simulink model "Task7"  (R2023b)
settings: Solver=VariableStepAuto  StartTime=0.0  StopTime=1800  RelTol=1e-3
InitFcn:
  | run("Linear_Model.m")
values from neighbouring files (symbols this model uses):
  A_Lat = [Yv   Yp+w0   Yr-u0         gravity*cos(theta0)     0 ... (first row only)    [Linear_Model.m]
  A_Long = [Xu                    Xw                        -w0                            -gravity*cos(theta0) ... (first row only)    [Linear_Model.m]
  B_Lat = [Yda          Ydr ... (first row only)    [Linear_Model.m]
  B_Long = [Xde                         Xdth ... (first row only)    [Linear_Model.m]
  C_Lat = eye(5)    [Linear_Model.m]
  C_Long = eye(4)    [Linear_Model.m]
  D_Lat = zeros(5,2)    [Linear_Model.m]
  D_Long = zeros(4,2)    [Linear_Model.m]
  F_gravity_0 = mass*gravity*[sin(states_0(8)) ... (first row only)    [Data_edit.m]
  gravity = Airplane_data(52)    [Data_edit.m]
  Ixx = Airplane_data(53)    [Data_edit.m]
  Iyy = Airplane_data(54)    [Data_edit.m]
  Izz = Airplane_data(55)    [Data_edit.m]
  M0 = [0;0;0]    [Data_edit.m]
  mass = Airplane_data(51)    [Data_edit.m]
  Matrix_controls = [ 0             Xde             Xdth            0 ... (first row only)    [Data_edit.m]
  Matrix_states = [Xu   0   Xw  0   0   0   0 ... (first row only)    [Data_edit.m]
  p0 = states_0(4)    [Data_edit.m]
  phi0 = states_0(7)    [Data_edit.m]
  psi0 = states_0(9)    [Data_edit.m]
  q0 = states_0(5)    [Data_edit.m]
  r0 = states_0(6)    [Data_edit.m]
  states_0 = Airplane_data(4:15)    [Data_edit.m]
  theta0 = states_0(8)    [Data_edit.m]
  u0 = states_0(1)    [Data_edit.m]
  v0 = states_0(2)    [Data_edit.m]
  w0 = states_0(3)    [Data_edit.m]
undefined symbols (not defined in the file or in its folder): Earth, sigbuilder_block, WGS84
libraries: simulink_extras x35, cstblocks x17, slpidlib x12, aerolibasang x2, aerolibfltsims x2, shared6dof x1, dspsigops x1, aerolibtransform2 x1
(part 2 of 2)

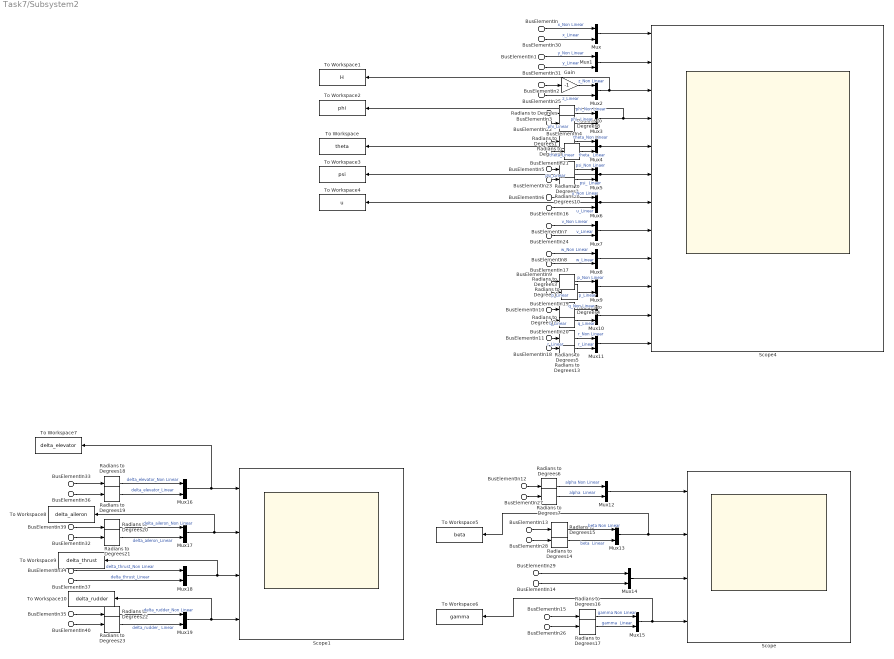
== system Task7/Subsystem2 ==
  BusElementIn16 : Inport  PortName=states_linear  Element=u
  BusElementIn17 : Inport  PortName=states_linear  Element=w
  BusElementIn18 : Inport  PortName=states_linear  Element=r
  BusElementIn19 : Inport  PortName=states_linear  Element=p
  BusElementIn20 : Inport  PortName=states_linear  Element=q
  BusElementIn21 : Inport  PortName=states_linear  Element=theta
  BusElementIn22 : Inport  PortName=states_linear  Element=phi
  BusElementIn23 : Inport  PortName=states_linear  Element=psi
  BusElementIn24 : Inport  PortName=states_linear  Element=v
  BusElementIn25 : Inport  PortName=states_linear  Element=H
  BusElementIn27 : Inport  PortName=states_linear  Element=alpha
  BusElementIn28 : Inport  PortName=states_linear  Element=beta
  BusElementIn29 : Inport  PortName=states_linear  Element=v_tot
  BusElementIn30 : Inport  PortName=states_linear  Element=x
  BusElementIn31 : Inport  PortName=states_linear  Element=y
  BusElementIn26 : Inport  PortName=states_linear  Element=gamma(rad)
  BusElementIn12 : Inport  Port=2  PortName=states  Element=alpha
  BusElementIn13 : Inport  Port=2  PortName=states  Element=betaa
  BusElementIn14 : Inport  Port=2  PortName=states  Element=v_tot
  BusElementIn : Inport  Port=2  PortName=states  Element=x
  BusElementIn1 : Inport  Port=2  PortName=states  Element=y
  BusElementIn2 : Inport  Port=2  PortName=states  Element=z
  BusElementIn3 : Inport  Port=2  PortName=states  Element=phi
  BusElementIn4 : Inport  Port=2  PortName=states  Element=ceta
  BusElementIn5 : Inport  Port=2  PortName=states  Element=psi
  BusElementIn6 : Inport  Port=2  PortName=states  Element=u
  BusElementIn7 : Inport  Port=2  PortName=states  Element=v
  BusElementIn8 : Inport  Port=2  PortName=states  Element=w
  BusElementIn9 : Inport  Port=2  PortName=states  Element=p
  BusElementIn10 : Inport  Port=2  PortName=states  Element=q
  BusElementIn11 : Inport  Port=2  PortName=states  Element=r
  BusElementIn15 : Inport  Port=2  PortName=states  Element=gamma
  BusElementIn32 : Inport  Port=3  PortName=Conrol Action Non Linear  Element=delta_aileron
  BusElementIn33 : Inport  Port=3  PortName=Conrol Action Non Linear  Element=delta_elevator
  BusElementIn34 : Inport  Port=3  PortName=Conrol Action Non Linear  Element=delta_thrust
  BusElementIn35 : Inport  Port=3  PortName=Conrol Action Non Linear  Element=delta_ruuder
  BusElementIn36 : Inport  Port=4  PortName="Conrol Action  Linear"  Element=Long_Control_Action.delta_elevator
  BusElementIn37 : Inport  Port=4  PortName="Conrol Action  Linear"  Element=Long_Control_Action.delta_thrust
  BusElementIn39 : Inport  Port=4  PortName="Conrol Action  Linear"  Element=Lat_Control_Action.delta_aileron
  BusElementIn40 : Inport  Port=4  PortName="Conrol Action  Linear"  Element=Lat_Control_Action.delta_ruuder
  Gain : Gain  Gain=-1
  Mux{,1..19} (20 alike) : Mux  Inputs=2
  Radians to Degrees{,1..23} (24 alike) : simulink_extras/Transformations/Radians to Degrees
  Scope : Scope  NumInputPorts=4
  Scope1 : Scope  NumInputPorts=4
  Scope4 : Scope  NumInputPorts=12
  To Workspace : ToWorkspace  VariableName=theta  SampleTime=-1
  To Workspace1 : ToWorkspace  VariableName=H  SampleTime=-1
  To Workspace10 : ToWorkspace  VariableName=delta_rudder  SampleTime=-1
  To Workspace2 : ToWorkspace  VariableName=phi  SampleTime=-1
  To Workspace3 : ToWorkspace  VariableName=psi  SampleTime=-1
  To Workspace4 : ToWorkspace  VariableName=u  SampleTime=-1
  To Workspace5 : ToWorkspace  VariableName=beta  SampleTime=-1
  To Workspace6 : ToWorkspace  VariableName=gamma  SampleTime=-1
  To Workspace7 : ToWorkspace  VariableName=delta_elevator  SampleTime=-1
  To Workspace8 : ToWorkspace  VariableName=delta_aileron  SampleTime=-1
  To Workspace9 : ToWorkspace  VariableName=delta_thrust  SampleTime=-1
  wires:
  BusElementIn1/1 -> Mux1/1  "y_Non Linear"
  BusElementIn/1 -> Mux/1  "x_Non Linear"
  Gain/1 -> Mux2/1  "z_Non Linear"
  BusElementIn2/1 -> Gain/1
  Mux/1 -> Scope4/1
  Mux1/1 -> Scope4/2
  Mux2/1 -> Scope4/3, To Workspace1/1
  BusElementIn4/1 -> Radians to Degrees1/1
  Radians to Degrees/1 -> Mux3/1  "phi_Non Linear"
  BusElementIn5/1 -> Radians to Degrees2/1
  Radians to Degrees1/1 -> Mux4/1  "theta_Non Linear"
  Radians to Degrees2/1 -> Mux5/1  "psi_Non Linaer"
  BusElementIn3/1 -> Radians to Degrees/1
  Mux5/1 -> To Workspace3/1, Scope4/6
  Mux4/1 -> To Workspace/1, Scope4/5
  Mux3/1 -> To Workspace2/1, Scope4/4
  Mux6/1 -> Scope4/7, To Workspace4/1
  Mux7/1 -> Scope4/8
  Mux8/1 -> Scope4/9
  BusElementIn6/1 -> Mux6/1  "u_Non Linear"
  BusElementIn7/1 -> Mux7/1  "v_Non Linear"
  BusElementIn8/1 -> Mux8/1  "w_Non Linear"
  Mux9/1 -> Scope4/10
  BusElementIn9/1 -> Radians to Degrees3/1
  Mux10/1 -> Scope4/11
  Mux11/1 -> Scope4/12
  BusElementIn10/1 -> Radians to Degrees4/1
  BusElementIn11/1 -> Radians to Degrees5/1
  Radians to Degrees3/1 -> Mux9/1  "p_Non Linear"
  Radians to Degrees4/1 -> Mux10/1  "q_Non Linear"
  Radians to Degrees5/1 -> Mux11/1  "r_Non Linear"
  BusElementIn30/1 -> Mux/2  "x_Linear"
  BusElementIn31/1 -> Mux1/2  "y_Linear"
  BusElementIn25/1 -> Mux2/2  "z_Linear"
  BusElementIn16/1 -> Mux6/2  "u_Linear"
  BusElementIn17/1 -> Mux8/2  "w_Linear"
  BusElementIn24/1 -> Mux7/2  "v_Linear"
  BusElementIn22/1 -> Radians to Degrees8/1  "phi_Linear"
  BusElementIn21/1 -> Radians to Degrees9/1  "theta_Linear"
  BusElementIn23/1 -> Radians to Degrees10/1  "psi_Linear"
  BusElementIn19/1 -> Radians to Degrees11/1  "p_Linear"
  BusElementIn20/1 -> Radians to Degrees12/1  "q_Linear"
  BusElementIn18/1 -> Radians to Degrees13/1  "r_Linear"
  Mux12/1 -> Scope/1
  BusElementIn12/1 -> Radians to Degrees6/1
  Radians to Degrees6/1 -> Mux12/1  "alpha Non Linear"
  Radians to Degrees7/1 -> Mux12/2  "alpha  Linear"
  BusElementIn27/1 -> Radians to Degrees7/1
  Mux13/1 -> To Workspace5/1, Scope/2
  Radians to Degrees8/1 -> Mux3/2  "phi_ Linear"
  Radians to Degrees9/1 -> Mux4/2  "theta_ Linear"
  Radians to Degrees10/1 -> Mux5/2  "psi_ Linaer"
  Radians to Degrees11/1 -> Mux9/2  "p_Linear"
  Radians to Degrees12/1 -> Mux10/2  "q_Linear"
  Radians to Degrees13/1 -> Mux11/2  "r_Linear"
  BusElementIn28/1 -> Radians to Degrees14/1
  Radians to Degrees14/1 -> Mux13/2  "beta  Linear"
  BusElementIn13/1 -> Radians to Degrees15/1
  Radians to Degrees15/1 -> Mux13/1  "beta Non Linear"
  Mux14/1 -> Scope/3
  BusElementIn14/1 -> Mux14/2
  BusElementIn29/1 -> Mux14/1
  BusElementIn15/1 -> Radians to Degrees16/1
  BusElementIn26/1 -> Radians to Degrees17/1
  Radians to Degrees16/1 -> Mux15/1  "gamma Non Linear"
  Radians to Degrees17/1 -> Mux15/2  "gamma  Linear"
  Mux16/1 -> To Workspace7/1, Scope1/1
  Mux17/1 -> To Workspace8/1, Scope1/2
  Mux18/1 -> To Workspace9/1, Scope1/3
  Mux19/1 -> To Workspace10/1, Scope1/4
  BusElementIn36/1 -> Radians to Degrees19/1
  BusElementIn33/1 -> Radians to Degrees18/1
  BusElementIn39/1 -> Radians to Degrees20/1
  BusElementIn32/1 -> Radians to Degrees21/1
  BusElementIn34/1 -> Mux18/1  "delta_thrust_Non Linear"
  BusElementIn37/1 -> Mux18/2  "delta_thrust_Linear"
  BusElementIn40/1 -> Radians to Degrees23/1
  BusElementIn35/1 -> Radians to Degrees22/1
  Radians to Degrees18/1 -> Mux16/1  "delta_elevator_Non Linear"
  Radians to Degrees19/1 -> Mux16/2  "delta_elevator_Linear"
  Radians to Degrees20/1 -> Mux17/1  "delta_aileron_Non Linear"
  Radians to Degrees21/1 -> Mux17/2  "delta_aileron_Linear"
  Radians to Degrees22/1 -> Mux19/1  "delta_rudder_Non Linear"
  Radians to Degrees23/1 -> Mux19/2  "delta_rudder_ Linear"
  Mux15/1 -> To Workspace6/1, Scope/4

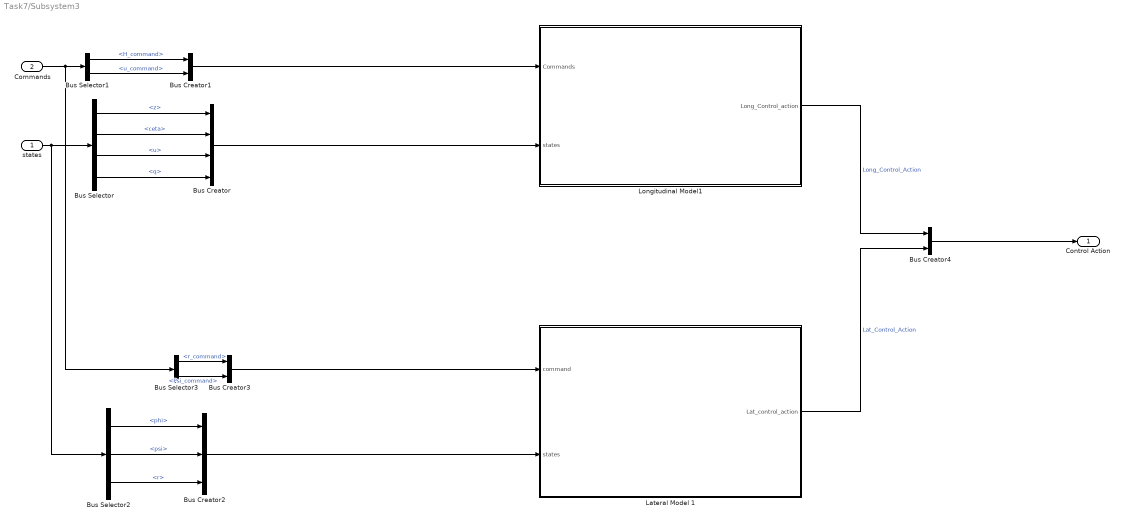
== system Task7/Subsystem3 ==
  states : Inport
  Commands : Inport  Port=2
  Bus Creator : BusCreator  Inputs=4
  Bus Creator1 : BusCreator  Inputs=2
  Bus Creator2 : BusCreator  Inputs=3
  Bus Creator3 : BusCreator  Inputs=2
  Bus Creator4 : BusCreator  Inputs=2
  Bus Selector : BusSelector  OutputSignals=z,ceta,u,q
  Bus Selector1 : BusSelector  OutputSignals=H_command,u_command
  Bus Selector2 : BusSelector  OutputSignals=phi,psi,r
  Bus Selector3 : BusSelector  OutputSignals=r_command,Psi_command
  Lateral Model 1 : Subsystem
  Longitudinal Model1 : Subsystem
  Control Action : Outport
  wires:
  states/1 -> Bus Selector2/1, Bus Selector/1
  Bus Selector/4 -> Bus Creator/4  "<q>"
  Bus Selector/3 -> Bus Creator/3  "<u>"
  Bus Selector/2 -> Bus Creator/2  "<ceta>"
  Bus Selector/1 -> Bus Creator/1  "<z>"
  Bus Creator/1 -> Longitudinal Model1/2(states)
  Commands/1 -> Bus Selector3/1, Bus Selector1/1
  Bus Selector1/1 -> Bus Creator1/1  "<H_command>"
  Bus Selector1/2 -> Bus Creator1/2  "<u_command>"
  Bus Creator1/1 -> Longitudinal Model1/1(Commands)
  Bus Selector2/1 -> Bus Creator2/1  "<phi>"
  Bus Selector2/2 -> Bus Creator2/2  "<psi>"
  Bus Selector2/3 -> Bus Creator2/3  "<r>"
  Bus Creator2/1 -> Lateral Model 1/2(states)
  Bus Creator3/1 -> Lateral Model 1/1(command)
  Bus Selector3/1 -> Bus Creator3/1  "<r_command>"
  Bus Selector3/2 -> Bus Creator3/2  "<Psi_command>"
  Longitudinal Model1/1(Long_Control_action) -> Bus Creator4/1  "Long_Control_Action"
  Lateral Model 1/1(Lat_control_action) -> Bus Creator4/2  "Lat_Control_Action"
  Bus Creator4/1 -> Control Action/1

== system Task7/Subsystem4 ==
  States : Inport
  Bus Selector1 : BusSelector  OutputSignals=x,y,z,phi,ceta,psi
  Demux : Demux  Outputs=2
  Flat Earth to LLA : aerolibtransform2/Flat Earth to LLA  units=Metric (MKS)  ptype=Earth (WGS84)  F=1/298.257223563  R=6378137  refPosPort=off  LL0=[0 10]  psi=0
  FlightGear Preconfigured 6DoF Animation : aerolibfltsims/FlightGear Preconfigured 6DoF Animation  xFlightGearVersion=v2019.1  DestinationIpAddress=127.0.0.1  DestinationPort=5502  SampleTime=1/30  packetVersion=24
  Generate Run Script : aerolibfltsims/Generate Run Script  Architecture=Win64  dataFlow=Send  GeometryModelName=c172p  AirportId=KSFO  RunwayId=10L  InitialAltitude=0  InitialHeading=0  OffsetDistance=0  OffsetAzimuth=0  InstallScenery=off  DisableShaders=on  OriginAddress=127.0.0.1  DestinationPort=5502  OriginPort=5505  LocalAddress=127.0.0.1  OutputFileName=runfg.bat  FlightGearBaseDirectory=C:\Program Files\FlightGear 2020.3
  Ground : Ground
  Mux : Mux  Inputs=3
  Mux1 : Mux  Inputs=3
  Mux2 : Mux
  wires:
  Mux1/1 -> Mux2/4
  Mux2/1 -> FlightGear Preconfigured 6DoF Animation/1
  Bus Selector1/6 -> Mux1/3  "<psi>"
  Flat Earth to LLA/1 -> Demux/1
  Bus Selector1/2 -> Mux/2  "<y>"
  Ground/1 -> Flat Earth to LLA/2
  Demux/1 -> Mux2/2
  Bus Selector1/5 -> Mux1/2  "<ceta>"
  Flat Earth to LLA/2 -> Mux2/3
  Mux/1 -> Flat Earth to LLA/1
  Bus Selector1/4 -> Mux1/1  "<phi>"
  Bus Selector1/3 -> Mux/3  "<z>"
  Bus Selector1/1 -> Mux/1  "<x>"
  Demux/2 -> Mux2/1
  States/1 -> Bus Selector1/1

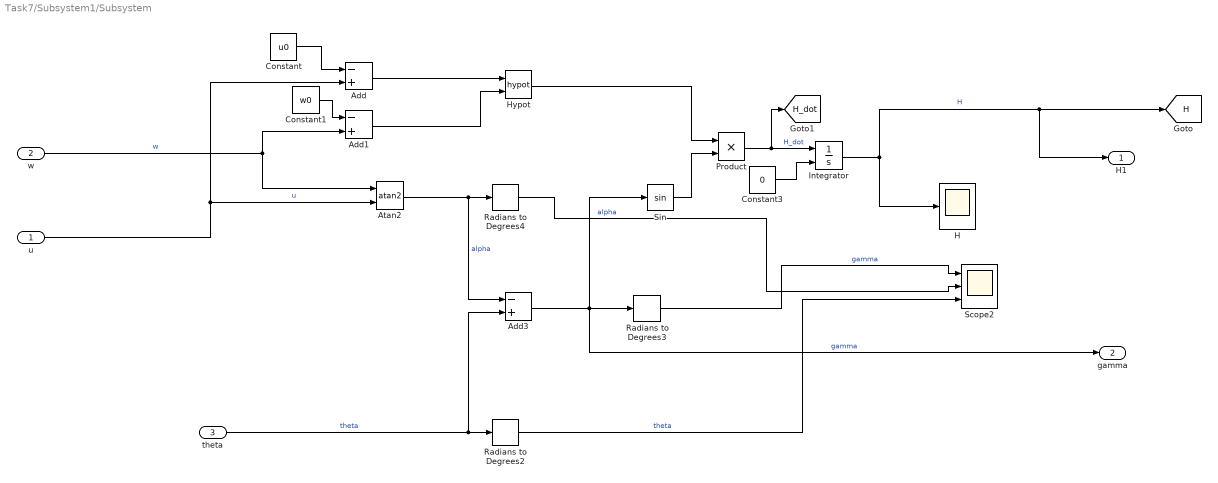
== system Task7/Subsystem1/Subsystem ==
  u : Inport
  w : Inport  Port=2
  theta : Inport  Port=3
  Add : Sum  Inputs=-+
  Add1 : Sum  Inputs=-+
  Add3 : Sum  Inputs=-+
  Atan2 : Trigonometry  Operator=atan2
  Constant : Constant  Value=u0
  Constant1 : Constant  Value=w0
  Constant3 : Constant  Value=0
  H : Scope
  Hypot : Math  Operator=hypot
  Integrator : Integrator  InitialConditionSource=external  InitialCondition=-states_0(12)
  Product : Product
  Radians to Degrees2 : simulink_extras/Transformations/Radians to Degrees
  Radians to Degrees3 : simulink_extras/Transformations/Radians to Degrees
  Radians to Degrees4 : simulink_extras/Transformations/Radians to Degrees
  Scope2 : Scope  NumInputPorts=3
  Sin : Trigonometry
  H1 : Outport
  gamma : Outport  Port=2
  tag scope: H=global, H_dot=global
  wires:
  Product/1 -> [H_dot], Integrator/1  "H_dot"
  Add3/1 -> gamma/1, Sin/1, Radians to Degrees3/1  "gamma"
  theta/1 -> Add3/2, Radians to Degrees2/1  "theta"
  Sin/1 -> Product/2
  Atan2/1 -> Radians to Degrees4/1, Add3/1  "alpha"
  Radians to Degrees4/1 -> Scope2/2  "alpha"
  Radians to Degrees2/1 -> Scope2/3  "theta"
  Radians to Degrees3/1 -> Scope2/1  "gamma"
  Integrator/1 -> H1/1, [H], H/1  "H"
  Hypot/1 -> Product/1
  Constant3/1 -> Integrator/2
  u/1 -> Add/2, Atan2/2  "u"
  w/1 -> Atan2/1, Add1/2  "w"
  Constant/1 -> Add/1
  Add/1 -> Hypot/1
  Constant1/1 -> Add1/1
  Add1/1 -> Hypot/2

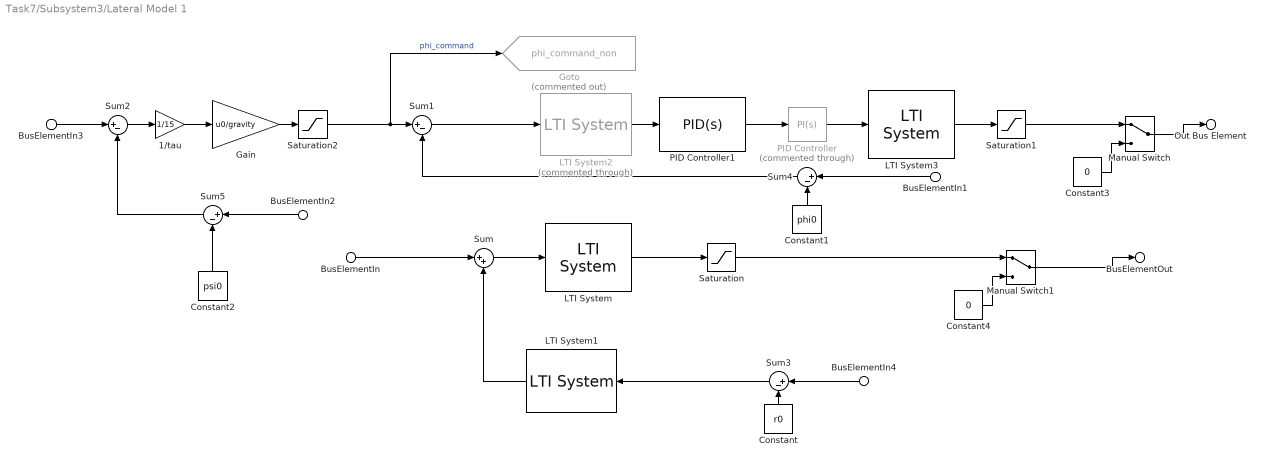
== system Task7/Subsystem3/Lateral Model 1 ==
  BusElementIn : Inport  PortName=command  Element=r_command
  BusElementIn3 : Inport  PortName=command  Element=Psi_command
  BusElementIn1 : Inport  Port=2  PortName=states  Element=phi
  BusElementIn2 : Inport  Port=2  PortName=states  Element=psi
  BusElementIn4 : Inport  Port=2  PortName=states  Element=r
  1/tau : Gain  Gain=1/15
  Constant : Constant  Value=r0
  Constant1 : Constant  Value=phi0
  Constant2 : Constant  Value=psi0
  Constant3 : Constant  Value=0
  Constant4 : Constant  Value=0
  Gain : Gain  Gain=u0/gravity
  Goto : Goto  Commented=on  GotoTag=phi_command_non  TagVisibility=global
  LTI System : cstblocks/LTI System  sys=servo  IC=[]  PadeOrder=0
  LTI System1 : cstblocks/LTI System  sys=HPF_Washout  IC=[]  PadeOrder=0
  LTI System2 : cstblocks/LTI System  Commented=through  sys=Roll_Comp  IC=[]  PadeOrder=0
  LTI System3 : cstblocks/LTI System  sys=servo  IC=[]  PadeOrder=0
  Manual Switch : ManualSwitch
  Manual Switch1 : ManualSwitch
  PID Controller : slpidlib/PID Controller  Commented=through  Controller=PI  Form=Parallel  TimeDomain=Continuous-time  UseExternalTs=off  SampleTime=-1  IntegratorMethod=Forward Euler  FilterMethod=Forward Euler  ControllerParametersSource=internal  P=1.6  I=.0254  UseKiTs=off  D=0  N=100  UseFilter=on  TunerSelectOption=Transfer Function Based (PID Tuner App)  InitialConditionSource=internal  InitialConditionForIntegrator=0  InitialConditionForFilter=0  DifferentiatorICPrevScaledInput=0  ExternalReset=none  TrackingMode=off  Kt=1  LimitOutput=off  SatLimitsSource=internal  UpperSaturationLimit=inf  LowerSaturationLimit=-inf  LinearizeAsGain=on  AntiWindupMode=none  Kb=1  LimitIntegrator=off  UpperIntegratorSaturationLimit=inf  LowerIntegratorSaturationLimit=-inf  POutMin=[]  POutMax=[]  IOutMin=[]  IOutMax=[]  DOutMin=[]  DOutMax=[]  NOutMin=[]  NOutMax=[]  SumOutMin=[]  SumOutMax=[]  SaturationOutMin=[]  SaturationOutMax=[]  PParamMin=[]  PParamMax=[]  IParamMin=[]  IParamMax=[]  DParamMin=[]  DParamMax=[]  NParamMin=[]  NParamMax=[]  KbParamMin=[]  KbParamMax=[]  KtParamMin=[]  KtParamMax=[]  KbOutMin=[]  KbOutMax=[]  KtOutMin=[]  KtOutMax=[]  IntegratorOutMin=[]  IntegratorOutMax=[]  FilterOutMin=[]  FilterOutMax=[]  SumI1OutMin=[]  SumI1OutMax=[]  SumI2OutMin=[]  SumI2OutMax=[]  SumI3OutMin=[]  SumI3OutMax=[]  SumI4OutMin=[]  SumI4OutMax=[]  SumDOutMin=[]  SumDOutMax=[]  DifferentiatorOutMin=[]  DifferentiatorOutMax=[]  FilterDiffOutCoefMin=[]  FilterDiffOutCoefMax=[]  ReciprocalOutMin=[]  ReciprocalOutMax=[]  SumDenOutMin=[]  SumDenOutMax=[]  SumNumOutMin=[]  SumNumOutMax=[]  DivideOutMin=[]  DivideOutMax=[]  UdiffTsProdOutMin=[]  UdiffTsProdOutMax=[]  NTsProdOutMin=[]  NTsProdOutMax=[]  UintegralTsProdOutMin=[]  UintegralTsProdOutMax=[]  UngainTsProdOutMin=[]  UngainTsProdOutMax=[]  ClampingZeroOutDataTypeStr=Inherit: Inherit via back propagation  ClampingZeroOutMin=[]  ClampingZeroOutMax=[]  FilterDenConstantOutDataTypeStr=Inherit: Inherit via back propagation  FilterDenConstantOutMin=[]  FilterDenConstantOutMax=[]  PCopyOutDataTypeStr=Inherit: Inherit via back propagation  PCopyOutMin=[]  PCopyOutMax=[]  NCopyOutDataTypeStr=Inherit: Inherit via back propagation  NCopyOutMin=[]  NCopyOutMax=[]  IntegratorContinuousStateAttributes=''  IntegratorStateMustResolveToSignalObject=off  IntegratorRTWStateStorageClass=Auto  FilterContinuousStateAttributes=''  FilterStateMustResolveToSignalObject=off  FilterRTWStateStorageClass=Auto  ParallelPVariant=InternalParameters  IdealPVariant=Disabled  IVariant=InternalParameters  DVariant=Disabled  IntegratorVariant=Continuous  SatVariant=Disabled  AWVariant=Passthrough  PCopyVariant=Disabled  TRVariant=Disabled  FdbkBlocksVariant=Forward  IdealPFdbkVariant=Disabled  SatFdbkVariant=Disabled  DerivativeFilterVariant=Disabled  NVariant=Disabled  NCopyVariant=Disabled_SignalSpec  FilterICVariant=Disabled  IntegratorICVariant=InternalICs  ExternalResetVariant=Disabled  TRSumVariant=Passthrough  SumFdbkVariant=Disabled  SumVariant=Sum_PI  TsampFilterVariant=InternalTs  TsampNgainVariant=Passthrough  TsampIntegralVariant=Disabled_SignalSpec  ExternalSaturationOutDataTypeStr=Inherit: Same as second input
  PID Controller1 : slpidlib/PID Controller  Controller=PID  Form=Parallel  TimeDomain=Continuous-time  UseExternalTs=off  SampleTime=-1  IntegratorMethod=Forward Euler  FilterMethod=Forward Euler  ControllerParametersSource=internal  P=3.4  I=0.05  UseKiTs=off  D=0.85  N=100  UseFilter=on  TunerSelectOption=Transfer Function Based (PID Tuner App)  InitialConditionSource=internal  InitialConditionForIntegrator=0  InitialConditionForFilter=0  DifferentiatorICPrevScaledInput=0  ExternalReset=none  TrackingMode=off  Kt=1  LimitOutput=off  SatLimitsSource=internal  UpperSaturationLimit=inf  LowerSaturationLimit=-inf  LinearizeAsGain=on  AntiWindupMode=none  Kb=1  LimitIntegrator=off  UpperIntegratorSaturationLimit=inf  LowerIntegratorSaturationLimit=-inf  POutMin=[]  POutMax=[]  IOutMin=[]  IOutMax=[]  DOutMin=[]  DOutMax=[]  NOutMin=[]  NOutMax=[]  SumOutMin=[]  SumOutMax=[]  SaturationOutMin=[]  SaturationOutMax=[]  PParamMin=[]  PParamMax=[]  IParamMin=[]  IParamMax=[]  DParamMin=[]  DParamMax=[]  NParamMin=[]  NParamMax=[]  KbParamMin=[]  KbParamMax=[]  KtParamMin=[]  KtParamMax=[]  KbOutMin=[]  KbOutMax=[]  KtOutMin=[]  KtOutMax=[]  IntegratorOutMin=[]  IntegratorOutMax=[]  FilterOutMin=[]  FilterOutMax=[]  SumI1OutMin=[]  SumI1OutMax=[]  SumI2OutMin=[]  SumI2OutMax=[]  SumI3OutMin=[]  SumI3OutMax=[]  SumI4OutMin=[]  SumI4OutMax=[]  SumDOutMin=[]  SumDOutMax=[]  DifferentiatorOutMin=[]  DifferentiatorOutMax=[]  FilterDiffOutCoefMin=[]  FilterDiffOutCoefMax=[]  ReciprocalOutMin=[]  ReciprocalOutMax=[]  SumDenOutMin=[]  SumDenOutMax=[]  SumNumOutMin=[]  SumNumOutMax=[]  DivideOutMin=[]  DivideOutMax=[]  UdiffTsProdOutMin=[]  UdiffTsProdOutMax=[]  NTsProdOutMin=[]  NTsProdOutMax=[]  UintegralTsProdOutMin=[]  UintegralTsProdOutMax=[]  UngainTsProdOutMin=[]  UngainTsProdOutMax=[]  ClampingZeroOutDataTypeStr=Inherit: Inherit via back propagation  ClampingZeroOutMin=[]  ClampingZeroOutMax=[]  FilterDenConstantOutDataTypeStr=Inherit: Inherit via back propagation  FilterDenConstantOutMin=[]  FilterDenConstantOutMax=[]  PCopyOutDataTypeStr=Inherit: Inherit via back propagation  PCopyOutMin=[]  PCopyOutMax=[]  NCopyOutDataTypeStr=Inherit: Inherit via back propagation  NCopyOutMin=[]  NCopyOutMax=[]  IntegratorContinuousStateAttributes=''  IntegratorStateMustResolveToSignalObject=off  IntegratorRTWStateStorageClass=Auto  FilterContinuousStateAttributes=''  FilterStateMustResolveToSignalObject=off  FilterRTWStateStorageClass=Auto  ParallelPVariant=InternalParameters  IdealPVariant=Disabled  IVariant=InternalParameters  DVariant=InternalParameters  IntegratorVariant=Continuous  SatVariant=Disabled  AWVariant=Passthrough  PCopyVariant=Disabled  TRVariant=Disabled  FdbkBlocksVariant=Forward  IdealPFdbkVariant=Disabled  SatFdbkVariant=Disabled  DerivativeFilterVariant=ContFilter  NVariant=InternalParameters  NCopyVariant=Disabled  FilterICVariant=InternalICsFilter  IntegratorICVariant=InternalICs  ExternalResetVariant=Disabled  TRSumVariant=Passthrough  SumFdbkVariant=Disabled  SumVariant=Sum_PID  TsampFilterVariant=InternalTs  TsampNgainVariant=Passthrough  TsampIntegralVariant=Disabled_SignalSpec  ExternalSaturationOutDataTypeStr=Inherit: Same as second input
  Saturation : Saturate  UpperLimit=deg2rad(30)  LowerLimit=deg2rad(-30)
  Saturation1 : Saturate  UpperLimit=deg2rad(50)  LowerLimit=deg2rad(-50)
  Saturation2 : Saturate  UpperLimit=deg2rad(30)  LowerLimit=deg2rad(-30)
  Sum : Sum  Inputs=|++
  Sum{1..5} (5 alike) : Sum  Inputs=|+-
  Out Bus Element : Outport  PortName=Lat_control_action  Element=delta_aileron
  BusElementOut : Outport  PortName=Lat_control_action  Element=delta_ruuder
  wires:
  Saturation2/1 -> Sum1/1, Goto/1  "phi_command"
  1/tau/1 -> Gain/1
  BusElementIn3/1 -> Sum2/1
  Sum2/1 -> 1/tau/1
  Gain/1 -> Saturation2/1
  Sum5/1 -> Sum2/2
  PID Controller1/1 -> PID Controller/1
  LTI System2/1 -> PID Controller1/1
  PID Controller/1 -> LTI System3/1
  LTI System3/1 -> Saturation1/1
  Sum1/1 -> LTI System2/1
  Sum4/1 -> Sum1/2
  LTI System1/1 -> Sum/2
  Sum3/1 -> LTI System1/1
  LTI System/1 -> Saturation/1
  Sum/1 -> LTI System/1
  BusElementIn/1 -> Sum/1
  Constant/1 -> Sum3/2
  BusElementIn1/1 -> Sum4/1
  Constant1/1 -> Sum4/2
  Constant2/1 -> Sum5/2
  BusElementIn4/1 -> Sum3/1
  BusElementIn2/1 -> Sum5/1
  Constant3/1 -> Manual Switch/2
  Saturation1/1 -> Manual Switch/1
  Manual Switch/1 -> Out Bus Element/1
  Constant4/1 -> Manual Switch1/2
  Saturation/1 -> Manual Switch1/1
  Manual Switch1/1 -> BusElementOut/1

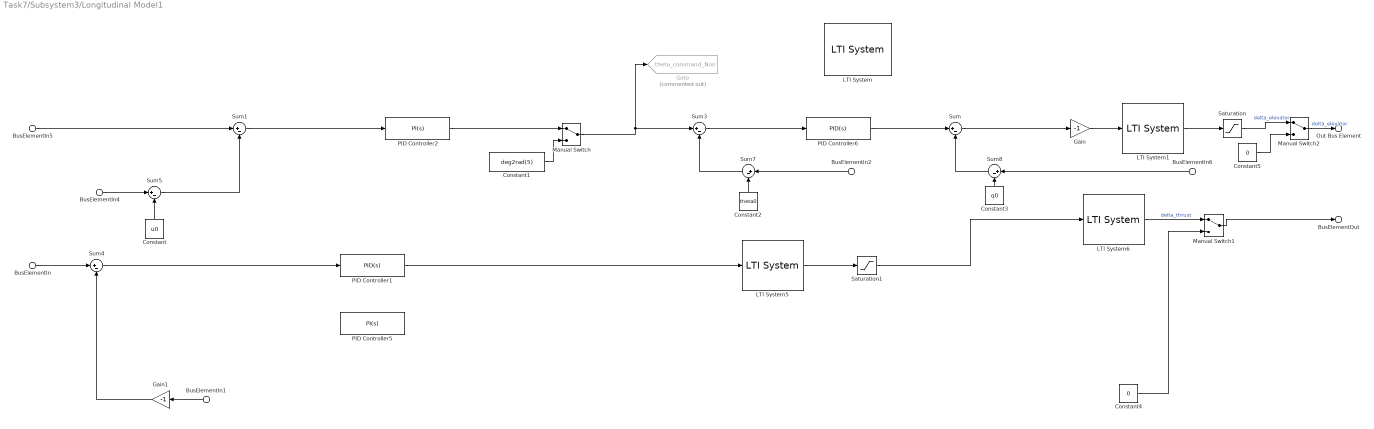
== system Task7/Subsystem3/Longitudinal Model1 ==
  BusElementIn5 : Inport  PortName=Commands  Element=u_command
  BusElementIn : Inport  PortName=Commands  Element=H_command
  BusElementIn1 : Inport  Port=2  PortName=states  Element=z
  BusElementIn4 : Inport  Port=2  PortName=states  Element=u
  BusElementIn2 : Inport  Port=2  PortName=states  Element=ceta
  BusElementIn6 : Inport  Port=2  PortName=states  Element=q
  Constant : Constant  Value=u0
  Constant1 : Constant  Value=deg2rad(5)
  Constant2 : Constant  Value=theta0
  Constant3 : Constant  Value=q0
  Constant4 : Constant  Value=0
  Constant5 : Constant  Value=0
  Gain : Gain  Gain=-1
  Gain1 : Gain  Gain=-1
  Goto : Goto  Commented=on  GotoTag=theta_command_Non  TagVisibility=global
  LTI System : cstblocks/LTI System  sys=PI_Pitch  IC=[]  PadeOrder=0
  LTI System1 : cstblocks/LTI System  sys=servo  IC=[]  PadeOrder=0
  LTI System5 : cstblocks/LTI System  sys=servo  IC=[]  PadeOrder=0
  LTI System6 : cstblocks/LTI System  sys=Engine_Lag  IC=[]  PadeOrder=0
  Manual Switch : ManualSwitch
  Manual Switch1 : ManualSwitch
  Manual Switch2 : ManualSwitch
  PID Controller1 : slpidlib/PID Controller  Controller=PID  Form=Parallel  TimeDomain=Continuous-time  UseExternalTs=off  SampleTime=-1  IntegratorMethod=Forward Euler  FilterMethod=Forward Euler  ControllerParametersSource=internal  P=88.8006309428434  I=0.0929360693607998  UseKiTs=off  D=2265.07533682159  N=14.0545983355681  UseFilter=on  TunerSelectOption=Transfer Function Based (PID Tuner App)  InitialConditionSource=internal  InitialConditionForIntegrator=0  InitialConditionForFilter=0  DifferentiatorICPrevScaledInput=0  ExternalReset=none  TrackingMode=off  Kt=1  LimitOutput=off  SatLimitsSource=internal  UpperSaturationLimit=inf  LowerSaturationLimit=-inf  LinearizeAsGain=on  AntiWindupMode=none  Kb=1  LimitIntegrator=off  UpperIntegratorSaturationLimit=inf  LowerIntegratorSaturationLimit=-inf  POutMin=[]  POutMax=[]  IOutMin=[]  IOutMax=[]  DOutMin=[]  DOutMax=[]  NOutMin=[]  NOutMax=[]  SumOutMin=[]  SumOutMax=[]  SaturationOutMin=[]  SaturationOutMax=[]  PParamMin=[]  PParamMax=[]  IParamMin=[]  IParamMax=[]  DParamMin=[]  DParamMax=[]  NParamMin=[]  NParamMax=[]  KbParamMin=[]  KbParamMax=[]  KtParamMin=[]  KtParamMax=[]  KbOutMin=[]  KbOutMax=[]  KtOutMin=[]  KtOutMax=[]  IntegratorOutMin=[]  IntegratorOutMax=[]  FilterOutMin=[]  FilterOutMax=[]  SumI1OutMin=[]  SumI1OutMax=[]  SumI2OutMin=[]  SumI2OutMax=[]  SumI3OutMin=[]  SumI3OutMax=[]  SumI4OutMin=[]  SumI4OutMax=[]  SumDOutMin=[]  SumDOutMax=[]  DifferentiatorOutMin=[]  DifferentiatorOutMax=[]  FilterDiffOutCoefMin=[]  FilterDiffOutCoefMax=[]  ReciprocalOutMin=[]  ReciprocalOutMax=[]  SumDenOutMin=[]  SumDenOutMax=[]  SumNumOutMin=[]  SumNumOutMax=[]  DivideOutMin=[]  DivideOutMax=[]  UdiffTsProdOutMin=[]  UdiffTsProdOutMax=[]  NTsProdOutMin=[]  NTsProdOutMax=[]  UintegralTsProdOutMin=[]  UintegralTsProdOutMax=[]  UngainTsProdOutMin=[]  UngainTsProdOutMax=[]  ClampingZeroOutDataTypeStr=Inherit: Inherit via back propagation  ClampingZeroOutMin=[]  ClampingZeroOutMax=[]  FilterDenConstantOutDataTypeStr=Inherit: Inherit via back propagation  FilterDenConstantOutMin=[]  FilterDenConstantOutMax=[]  PCopyOutDataTypeStr=Inherit: Inherit via back propagation  PCopyOutMin=[]  PCopyOutMax=[]  NCopyOutDataTypeStr=Inherit: Inherit via back propagation  NCopyOutMin=[]  NCopyOutMax=[]  IntegratorContinuousStateAttributes=''  IntegratorStateMustResolveToSignalObject=off  IntegratorRTWStateStorageClass=Auto  FilterContinuousStateAttributes=''  FilterStateMustResolveToSignalObject=off  FilterRTWStateStorageClass=Auto  ParallelPVariant=InternalParameters  IdealPVariant=Disabled  IVariant=InternalParameters  DVariant=InternalParameters  IntegratorVariant=Continuous  SatVariant=Disabled  AWVariant=Passthrough  PCopyVariant=Disabled  TRVariant=Disabled  FdbkBlocksVariant=Forward  IdealPFdbkVariant=Disabled  SatFdbkVariant=Disabled  DerivativeFilterVariant=ContFilter  NVariant=InternalParameters  NCopyVariant=Disabled  FilterICVariant=InternalICsFilter  IntegratorICVariant=InternalICs  ExternalResetVariant=Disabled  TRSumVariant=Passthrough  SumFdbkVariant=Disabled  SumVariant=Sum_PID  TsampFilterVariant=InternalTs  TsampNgainVariant=Passthrough  TsampIntegralVariant=Disabled_SignalSpec  ExternalSaturationOutDataTypeStr=Inherit: Same as second input
  PID Controller2 : slpidlib/PID Controller  Controller=PI  Form=Parallel  TimeDomain=Continuous-time  UseExternalTs=off  SampleTime=-1  IntegratorMethod=Forward Euler  FilterMethod=Forward Euler  ControllerParametersSource=internal  P=-0.0029780732187298  I=-6.00662195955179e-05  UseKiTs=off  D=-0.0901078465434796  N=4.30153629977803  UseFilter=on  TunerSelectOption=Transfer Function Based (PID Tuner App)  InitialConditionSource=internal  InitialConditionForIntegrator=0  InitialConditionForFilter=0  DifferentiatorICPrevScaledInput=0  ExternalReset=none  TrackingMode=off  Kt=1  LimitOutput=off  SatLimitsSource=internal  UpperSaturationLimit=inf  LowerSaturationLimit=-inf  LinearizeAsGain=on  AntiWindupMode=none  Kb=1  LimitIntegrator=off  UpperIntegratorSaturationLimit=inf  LowerIntegratorSaturationLimit=-inf  POutMin=[]  POutMax=[]  IOutMin=[]  IOutMax=[]  DOutMin=[]  DOutMax=[]  NOutMin=[]  NOutMax=[]  SumOutMin=[]  SumOutMax=[]  SaturationOutMin=[]  SaturationOutMax=[]  PParamMin=[]  PParamMax=[]  IParamMin=[]  IParamMax=[]  DParamMin=[]  DParamMax=[]  NParamMin=[]  NParamMax=[]  KbParamMin=[]  KbParamMax=[]  KtParamMin=[]  KtParamMax=[]  KbOutMin=[]  KbOutMax=[]  KtOutMin=[]  KtOutMax=[]  IntegratorOutMin=[]  IntegratorOutMax=[]  FilterOutMin=[]  FilterOutMax=[]  SumI1OutMin=[]  SumI1OutMax=[]  SumI2OutMin=[]  SumI2OutMax=[]  SumI3OutMin=[]  SumI3OutMax=[]  SumI4OutMin=[]  SumI4OutMax=[]  SumDOutMin=[]  SumDOutMax=[]  DifferentiatorOutMin=[]  DifferentiatorOutMax=[]  FilterDiffOutCoefMin=[]  FilterDiffOutCoefMax=[]  ReciprocalOutMin=[]  ReciprocalOutMax=[]  SumDenOutMin=[]  SumDenOutMax=[]  SumNumOutMin=[]  SumNumOutMax=[]  DivideOutMin=[]  DivideOutMax=[]  UdiffTsProdOutMin=[]  UdiffTsProdOutMax=[]  NTsProdOutMin=[]  NTsProdOutMax=[]  UintegralTsProdOutMin=[]  UintegralTsProdOutMax=[]  UngainTsProdOutMin=[]  UngainTsProdOutMax=[]  ClampingZeroOutDataTypeStr=Inherit: Inherit via back propagation  ClampingZeroOutMin=[]  ClampingZeroOutMax=[]  FilterDenConstantOutDataTypeStr=Inherit: Inherit via back propagation  FilterDenConstantOutMin=[]  FilterDenConstantOutMax=[]  PCopyOutDataTypeStr=Inherit: Inherit via back propagation  PCopyOutMin=[]  PCopyOutMax=[]  NCopyOutDataTypeStr=Inherit: Inherit via back propagation  NCopyOutMin=[]  NCopyOutMax=[]  IntegratorContinuousStateAttributes=''  IntegratorStateMustResolveToSignalObject=off  IntegratorRTWStateStorageClass=Auto  FilterContinuousStateAttributes=''  FilterStateMustResolveToSignalObject=off  FilterRTWStateStorageClass=Auto  ParallelPVariant=InternalParameters  IdealPVariant=Disabled  IVariant=InternalParameters  DVariant=Disabled  IntegratorVariant=Continuous  SatVariant=Disabled  AWVariant=Passthrough  PCopyVariant=Disabled  TRVariant=Disabled  FdbkBlocksVariant=Forward  IdealPFdbkVariant=Disabled  SatFdbkVariant=Disabled  DerivativeFilterVariant=Disabled  NVariant=Disabled  NCopyVariant=Disabled_SignalSpec  FilterICVariant=Disabled  IntegratorICVariant=InternalICs  ExternalResetVariant=Disabled  TRSumVariant=Passthrough  SumFdbkVariant=Disabled  SumVariant=Sum_PI  TsampFilterVariant=InternalTs  TsampNgainVariant=Passthrough  TsampIntegralVariant=Disabled_SignalSpec  ExternalSaturationOutDataTypeStr=Inherit: Same as second input
  PID Controller5 : slpidlib/PID Controller  Controller=PI  Form=Parallel  TimeDomain=Continuous-time  UseExternalTs=off  SampleTime=-1  IntegratorMethod=Forward Euler  FilterMethod=Forward Euler  ControllerParametersSource=internal  P=114.381280532238  I=0.143547769881875  UseKiTs=off  D=25000  N=100  UseFilter=on  TunerSelectOption=Transfer Function Based (PID Tuner App)  InitialConditionSource=internal  InitialConditionForIntegrator=0  InitialConditionForFilter=0  DifferentiatorICPrevScaledInput=0  ExternalReset=none  TrackingMode=off  Kt=1  LimitOutput=off  SatLimitsSource=internal  UpperSaturationLimit=inf  LowerSaturationLimit=-inf  LinearizeAsGain=on  AntiWindupMode=none  Kb=1  LimitIntegrator=off  UpperIntegratorSaturationLimit=inf  LowerIntegratorSaturationLimit=-inf  POutMin=[]  POutMax=[]  IOutMin=[]  IOutMax=[]  DOutMin=[]  DOutMax=[]  NOutMin=[]  NOutMax=[]  SumOutMin=[]  SumOutMax=[]  SaturationOutMin=[]  SaturationOutMax=[]  PParamMin=[]  PParamMax=[]  IParamMin=[]  IParamMax=[]  DParamMin=[]  DParamMax=[]  NParamMin=[]  NParamMax=[]  KbParamMin=[]  KbParamMax=[]  KtParamMin=[]  KtParamMax=[]  KbOutMin=[]  KbOutMax=[]  KtOutMin=[]  KtOutMax=[]  IntegratorOutMin=[]  IntegratorOutMax=[]  FilterOutMin=[]  FilterOutMax=[]  SumI1OutMin=[]  SumI1OutMax=[]  SumI2OutMin=[]  SumI2OutMax=[]  SumI3OutMin=[]  SumI3OutMax=[]  SumI4OutMin=[]  SumI4OutMax=[]  SumDOutMin=[]  SumDOutMax=[]  DifferentiatorOutMin=[]  DifferentiatorOutMax=[]  FilterDiffOutCoefMin=[]  FilterDiffOutCoefMax=[]  ReciprocalOutMin=[]  ReciprocalOutMax=[]  SumDenOutMin=[]  SumDenOutMax=[]  SumNumOutMin=[]  SumNumOutMax=[]  DivideOutMin=[]  DivideOutMax=[]  UdiffTsProdOutMin=[]  UdiffTsProdOutMax=[]  NTsProdOutMin=[]  NTsProdOutMax=[]  UintegralTsProdOutMin=[]  UintegralTsProdOutMax=[]  UngainTsProdOutMin=[]  UngainTsProdOutMax=[]  ClampingZeroOutDataTypeStr=Inherit: Inherit via back propagation  ClampingZeroOutMin=[]  ClampingZeroOutMax=[]  FilterDenConstantOutDataTypeStr=Inherit: Inherit via back propagation  FilterDenConstantOutMin=[]  FilterDenConstantOutMax=[]  PCopyOutDataTypeStr=Inherit: Inherit via back propagation  PCopyOutMin=[]  PCopyOutMax=[]  NCopyOutDataTypeStr=Inherit: Inherit via back propagation  NCopyOutMin=[]  NCopyOutMax=[]  IntegratorContinuousStateAttributes=''  IntegratorStateMustResolveToSignalObject=off  IntegratorRTWStateStorageClass=Auto  FilterContinuousStateAttributes=''  FilterStateMustResolveToSignalObject=off  FilterRTWStateStorageClass=Auto  ParallelPVariant=InternalParameters  IdealPVariant=Disabled  IVariant=InternalParameters  DVariant=Disabled  IntegratorVariant=Continuous  SatVariant=Disabled  AWVariant=Passthrough  PCopyVariant=Disabled  TRVariant=Disabled  FdbkBlocksVariant=Forward  IdealPFdbkVariant=Disabled  SatFdbkVariant=Disabled  DerivativeFilterVariant=Disabled  NVariant=Disabled  NCopyVariant=Disabled_SignalSpec  FilterICVariant=Disabled  IntegratorICVariant=InternalICs  ExternalResetVariant=Disabled  TRSumVariant=Passthrough  SumFdbkVariant=Disabled  SumVariant=Sum_PI  TsampFilterVariant=InternalTs  TsampNgainVariant=Passthrough  TsampIntegralVariant=Disabled_SignalSpec  ExternalSaturationOutDataTypeStr=Inherit: Same as second input
  PID Controller6 : slpidlib/PID Controller  Controller=PID  Form=Parallel  TimeDomain=Continuous-time  UseExternalTs=off  SampleTime=-1  IntegratorMethod=Forward Euler  FilterMethod=Forward Euler  ControllerParametersSource=internal  P=3.70277868694912  I=0.831149312790549  UseKiTs=off  D=1.48691502004034  N=20.9794311620465  UseFilter=on  TunerSelectOption=Transfer Function Based (PID Tuner App)  InitialConditionSource=internal  InitialConditionForIntegrator=0  InitialConditionForFilter=0  DifferentiatorICPrevScaledInput=0  ExternalReset=none  TrackingMode=off  Kt=1  LimitOutput=off  SatLimitsSource=internal  UpperSaturationLimit=inf  LowerSaturationLimit=-inf  LinearizeAsGain=on  AntiWindupMode=none  Kb=1  LimitIntegrator=off  UpperIntegratorSaturationLimit=inf  LowerIntegratorSaturationLimit=-inf  POutMin=[]  POutMax=[]  IOutMin=[]  IOutMax=[]  DOutMin=[]  DOutMax=[]  NOutMin=[]  NOutMax=[]  SumOutMin=[]  SumOutMax=[]  SaturationOutMin=[]  SaturationOutMax=[]  PParamMin=[]  PParamMax=[]  IParamMin=[]  IParamMax=[]  DParamMin=[]  DParamMax=[]  NParamMin=[]  NParamMax=[]  KbParamMin=[]  KbParamMax=[]  KtParamMin=[]  KtParamMax=[]  KbOutMin=[]  KbOutMax=[]  KtOutMin=[]  KtOutMax=[]  IntegratorOutMin=[]  IntegratorOutMax=[]  FilterOutMin=[]  FilterOutMax=[]  SumI1OutMin=[]  SumI1OutMax=[]  SumI2OutMin=[]  SumI2OutMax=[]  SumI3OutMin=[]  SumI3OutMax=[]  SumI4OutMin=[]  SumI4OutMax=[]  SumDOutMin=[]  SumDOutMax=[]  DifferentiatorOutMin=[]  DifferentiatorOutMax=[]  FilterDiffOutCoefMin=[]  FilterDiffOutCoefMax=[]  ReciprocalOutMin=[]  ReciprocalOutMax=[]  SumDenOutMin=[]  SumDenOutMax=[]  SumNumOutMin=[]  SumNumOutMax=[]  DivideOutMin=[]  DivideOutMax=[]  UdiffTsProdOutMin=[]  UdiffTsProdOutMax=[]  NTsProdOutMin=[]  NTsProdOutMax=[]  UintegralTsProdOutMin=[]  UintegralTsProdOutMax=[]  UngainTsProdOutMin=[]  UngainTsProdOutMax=[]  ClampingZeroOutDataTypeStr=Inherit: Inherit via back propagation  ClampingZeroOutMin=[]  ClampingZeroOutMax=[]  FilterDenConstantOutDataTypeStr=Inherit: Inherit via back propagation  FilterDenConstantOutMin=[]  FilterDenConstantOutMax=[]  PCopyOutDataTypeStr=Inherit: Inherit via back propagation  PCopyOutMin=[]  PCopyOutMax=[]  NCopyOutDataTypeStr=Inherit: Inherit via back propagation  NCopyOutMin=[]  NCopyOutMax=[]  IntegratorContinuousStateAttributes=''  IntegratorStateMustResolveToSignalObject=off  IntegratorRTWStateStorageClass=Auto  FilterContinuousStateAttributes=''  FilterStateMustResolveToSignalObject=off  FilterRTWStateStorageClass=Auto  ParallelPVariant=InternalParameters  IdealPVariant=Disabled  IVariant=InternalParameters  DVariant=InternalParameters  IntegratorVariant=Continuous  SatVariant=Disabled  AWVariant=Passthrough  PCopyVariant=Disabled  TRVariant=Disabled  FdbkBlocksVariant=Forward  IdealPFdbkVariant=Disabled  SatFdbkVariant=Disabled  DerivativeFilterVariant=ContFilter  NVariant=InternalParameters  NCopyVariant=Disabled  FilterICVariant=InternalICsFilter  IntegratorICVariant=InternalICs  ExternalResetVariant=Disabled  TRSumVariant=Passthrough  SumFdbkVariant=Disabled  SumVariant=Sum_PID  TsampFilterVariant=InternalTs  TsampNgainVariant=Passthrough  TsampIntegralVariant=Disabled_SignalSpec  ExternalSaturationOutDataTypeStr=Inherit: Same as second input
  Saturation : Saturate  UpperLimit=deg2rad(25)  LowerLimit=deg2rad(-25)
  Saturation1 : Saturate  UpperLimit=65369  LowerLimit=-269369.84
  Sum{,1,3..5,7..8} (7 alike) : Sum  Inputs=|+-
  Out Bus Element : Outport  PortName=Long_Control_action  Element=delta_elevator
  BusElementOut : Outport  PortName=Long_Control_action  Element=delta_thrust
  wires:
  Manual Switch/1 -> Sum3/1, Goto/1
  Sum1/1 -> PID Controller2/1
  BusElementIn5/1 -> Sum1/1
  PID Controller1/1 -> LTI System5/1
  Sum4/1 -> PID Controller1/1
  Saturation1/1 -> LTI System6/1
  LTI System5/1 -> Saturation1/1
  BusElementIn/1 -> Sum4/1
  Sum7/1 -> Sum3/2
  Sum5/1 -> Sum1/2
  Sum3/1 -> PID Controller6/1
  PID Controller6/1 -> Sum/1
  Sum/1 -> Gain/1
  Gain/1 -> LTI System1/1
  LTI System1/1 -> Saturation/1
  Constant/1 -> Sum5/2
  BusElementIn2/1 -> Sum7/1
  Constant2/1 -> Sum7/2
  Sum8/1 -> Sum/2
  Constant3/1 -> Sum8/2
  BusElementIn1/1 -> Gain1/1
  Gain1/1 -> Sum4/2
  BusElementIn4/1 -> Sum5/1
  BusElementIn6/1 -> Sum8/1
  Constant1/1 -> Manual Switch/2
  PID Controller2/1 -> Manual Switch/1
  Constant4/1 -> Manual Switch1/2
  LTI System6/1 -> Manual Switch1/1  "delta_thrust"
  Manual Switch1/1 -> BusElementOut/1
  Manual Switch2/1 -> Out Bus Element/1  "delta_elevator"
  Saturation/1 -> Manual Switch2/1  "delta_elevator"
  Constant5/1 -> Manual Switch2/2

== matlab function Task7/Subsystem1/MATLAB Function ==
  data: velocity input; x_dot output; angles input; y_dot output; z_dot output
function [x_dot,y_dot,z_dot] = fcn(velocity,angles)

u=velocity(1);
v=velocity(2);
w=velocity(3);
phi=angles(1);
theta=angles(2);
psi=angles(3);
XYZ=eul2rotm([psi,theta,phi])*[u;v;w];
x_dot=XYZ(1);
y_dot=XYZ(2);
z_dot=XYZ(3);
